simulink library "create_EB"  (R2018b)
settings: Solver=ode45  StartTime=0.0  StopTime=10.0  RelTol=1e-3  EnableMultiTasking=on
libraries: carnot x1
settings Model: Creator=lena.frank  LastModifiedBy=P41573
settings DataIOCC: LimitDataPoints=on  SaveFormat=Array  SignalLoggingSaveFormat=ModelDataLogs
settings OptimizationCC: ExpressionDepthLimit=2147483647  LifeSpan=inf
settings DebuggingCC: UnderspecifiedInitializationDetection=Classic  MergeDetectMultiDrivingBlocksExec=none  SolverPrmCheckMsg=warning  FcnCallInpInsideContextMsg=warning  StateNameClashWarn=warning  SFUnexpectedBacktrackingDiag=warning  SFNoUnconditionalDefaultTransitionDiag=warning  SFExecutionAtInitializationDiag=none
settings HardwareCC: ProdBitPerPointer=32  ProdBitPerSizeT=32  ProdBitPerPtrDiffT=32  ProdLargestAtomicFloat=None  ProdIntDivRoundTo=Undefined  ProdEndianess=Unspecified  ProdWordSize=32  ProdHWDeviceType=32-bit Generic
settings ModelReferenceCC: PropagateSignalLabelsOutOfModel=off
settings SFSimCC: SimUseLocalCustomCode=off
settings RTWCC: RTWUseLocalCustomCode=off
settings CodeAppCC: StateflowObjectComments=on
settings GRTTargetCC: TargetLangStandard=C89/C90 (ANSI)  GeneratePreprocessorConditionals=Disable all  CombineOutputUpdateFcns=off  GRTInterface=on
settings ConfigComp: CovMetricSettings=dw  CovHtmlReporting=on  CovSaveCumulativeToWorkspaceVar=on  CovSaveSingleToWorkspaceVar=on  CovExternalEMLEnable=off

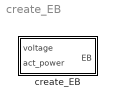
== system create_EB ==
  create_EB : Subsystem  mask(create EB){eID=Power only, f=50, pf1=1, pf2=1, pf3=1}
      mask prompts: eID "ID for electric calculation"; f "frequency [Hz]"; pf1 "power factor line 1 [1]"; pf2 "power factor line 2 [1]"; pf3 "power factor line 3 [1]"
      mask help: Block to create an EB with the variable inputs ActivePower and Voltage. The other values can be set as constants in the mask.
      mask Help: web(fullfile(path_carnot('help'),'create_EB.html'),'-helpbrowser')
      mask TypeOptions eID: basic_create_EB/eID
      mask TypeOptions f: basic_create_EB/f
      mask TypeOptions pf1: basic_create_EB/pf1
      mask TypeOptions pf2: basic_create_EB/pf2
      mask TypeOptions pf3: basic_create_EB/pf3

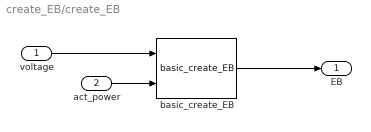
== system create_EB/create_EB ==
  voltage : Inport
  act_power : Inport  Port=2
  basic_create_EB : carnot/Basic/Electric/basic_create_EB  eID=Power only  f=f  pf1=pf1  pf2=pf2  pf3=pf3
      settings: SourceProductName=Carnot
  EB : Outport
  wires:
  voltage/1 -> basic_create_EB/1
  act_power/1 -> basic_create_EB/2
  basic_create_EB/1 -> EB/1
